simulink model "LKAS_with_MPC"  (R2021b)
settings: Solver=FixedStepAuto  StartTime=0.0  StopTime=20  FixedStep=0.1  MinStep=0.001  RelTol=1e-3
PostLoadFcn:
  | if exist('scenarioName','var')
  |   helperAEBSetUp(scenarioName)
  | else
  |   helperAEBSetUp()
  | end
undefined symbols (not defined in the file): A, B, C, D, Vx_const, X0, Y0, Yaw0
libraries: mpclib x1, drivingscenarioandsensors x1
CloseFcn:
  | helperAEBSetUp(true);
settings Model: Creator=user  LastModifiedBy=user
settings DataIOCC: SaveFormat=Array  SaveState=on

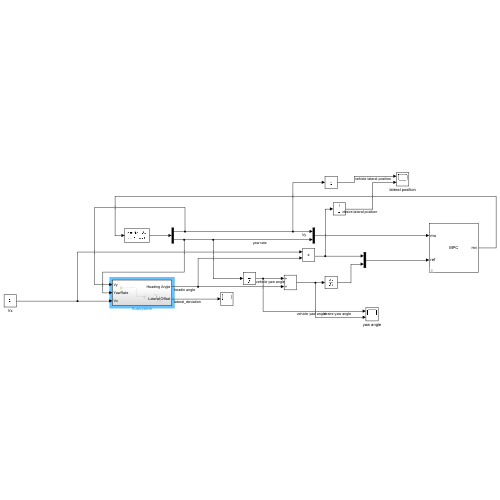
[thumbnail: Simulink's stored preview of the top-level diagram]
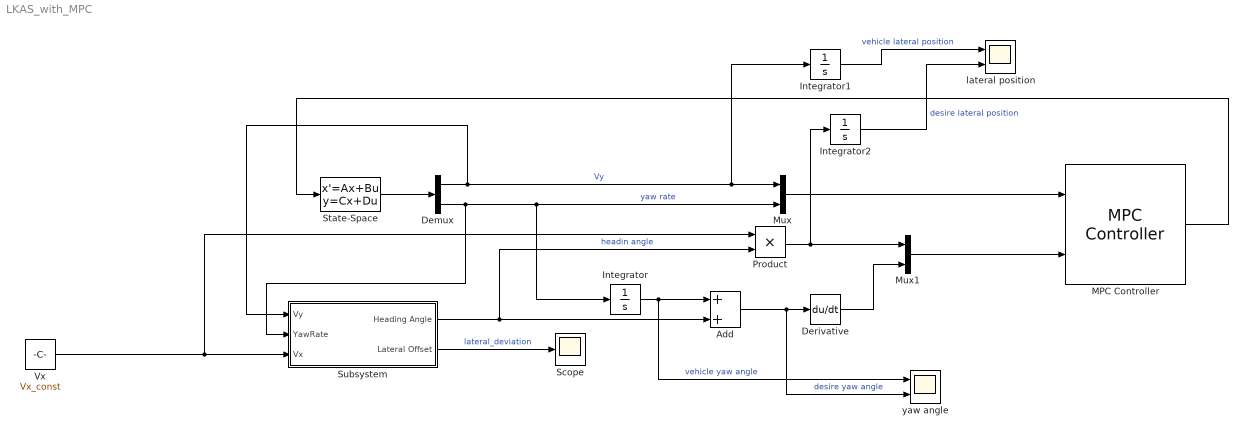
== system LKAS_with_MPC ==
  Add : Sum
  Demux : Demux  Outputs=2
  Derivative : Derivative
  Integrator : Integrator  InitialCondition=Yaw0
  Integrator1 : Integrator
  Integrator2 : Integrator
  MPC Controller : mpclib/MPC Controller  SCDEnableBlockLinearizationSpecification=on  mpcobj=mpc1  is_multiple=0  enable_value=0  return_u0=off  updateMPCinCallerWorkspace=on  md_inport=off  mv_inport=off  uref_inport=off  return_cost=off  return_mvseq=off  return_qpstatus=off  return_xseq=off  return_state=off  return_ovseq=off  state_inport=off  umin_inport=off  umax_inport=off  ymin_inport=off  ymax_inport=off  cc_inport=off  ywt_inport=off  uwt_inport=off  duwt_inport=off  rhoeps_inport=off  pm_inport=off  MaximumP=10  HorizonChoice=FixedHorizon  n_ts=0.1  n_p=20  n_mv=1  n_md=0  n_ud=0  n_mo=2  n_uo=0  BlockDataType=double  SampleTimeInherited=off  switch_inport=off
  Mux : Mux  Inputs=2
  Mux1 : Mux  Inputs=2
  Product : Product
  Scope : Scope
  State-Space : StateSpace  A=A  B=B  C=C  D=D  InitialCondition=0
  Subsystem : Subsystem
  Vx : Constant  Value=Vx_const
  lateral position : Scope  NumInputPorts=2
  yaw angle : Scope  NumInputPorts=2
  wires:
  Vx/1 -> Product/1, Subsystem/3(Vx)
  MPC Controller/1 -> State-Space/1
  Subsystem/1(Heading Angle) -> Product/2, Add/2  "headin angle"
  Integrator/1 -> yaw angle/1, Add/1  "vehicle yaw angle"
  Add/1 -> yaw angle/2, Derivative/1  "desire yaw angle"
  Mux1/1 -> MPC Controller/2
  Derivative/1 -> Mux1/2
  Subsystem/2(Lateral Offset) -> Scope/1  "lateral_deviation"
  Product/1 -> Integrator2/1, Mux1/1
  Mux/1 -> MPC Controller/1
  Demux/1 -> Integrator1/1, Mux/1, Subsystem/1(Vy)  "Vy"
  Demux/2 -> Subsystem/2(YawRate), Mux/2, Integrator/1  "yaw rate"
  State-Space/1 -> Demux/1
  Integrator1/1 -> lateral position/1  "vehicle lateral position"
  Integrator2/1 -> lateral position/2  "desire lateral position"

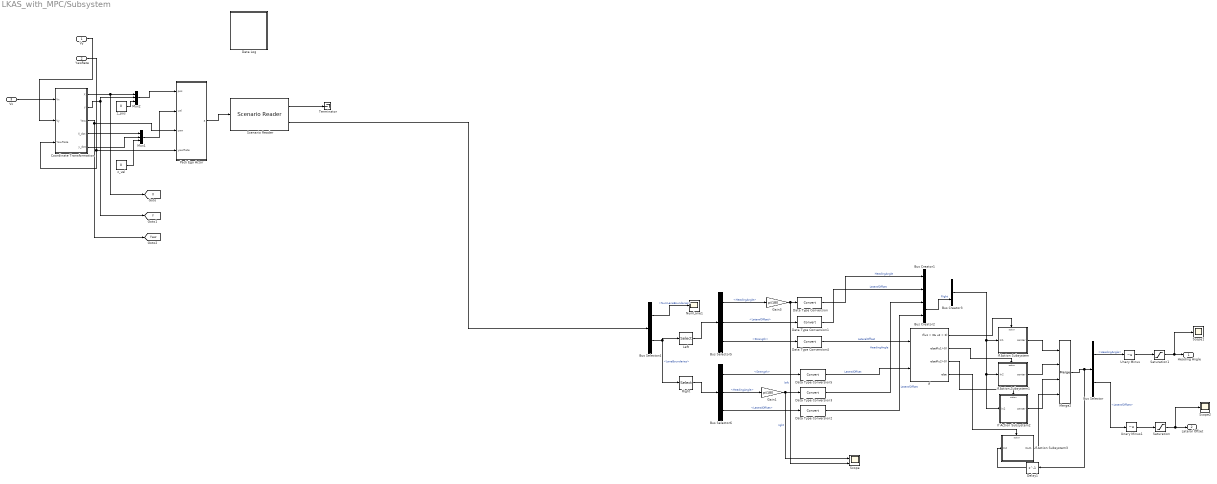
== system LKAS_with_MPC/Subsystem ==
  Vy : Inport
  YawRate : Inport  Port=2
  Vx : Inport  Port=3
  Bus Creator1 : BusCreator  Inputs=2
  Bus Creator2 : BusCreator  Inputs=2
  Bus Creator3 : BusCreator  Inputs=2
  Bus Selector : BusSelector  OutputSignals=HeadingAngle,LateralOffset
  Bus Selector4 : BusSelector  OutputSignals=NumLaneBoundaries,LaneBoundaries
  Bus Selector5 : BusSelector  OutputSignals=HeadingAngle,LateralOffset,Strength
  Bus Selector6 : BusSelector  OutputSignals=Strength,HeadingAngle,LateralOffset
  Coordinate Transformation : Subsystem
  Data Log : Subsystem
  Data Type Conversion{,1..5} (6 alike) : DataTypeConversion
  Delay1 : Delay  DelayLength=1
  Gain1 : Gain  Gain=pi/180
  Gain3 : Gain  Gain=pi/180
  If : If  NumInputs=2  IfExpression=u1 > 0& u2 > 0  ElseIfExpressions=u1>0, u2>0
  If Action Subsystem : Subsystem  TreatAsAtomicUnit=on
  If Action Subsystem1 : Subsystem  TreatAsAtomicUnit=on
  If Action Subsystem2 : Subsystem  TreatAsAtomicUnit=on
  If Action Subsystem3 : Subsystem  TreatAsAtomicUnit=on
  Left : Selector  InputPortWidth=2  IndexOptions=Index vector (dialog)  Indices=[1]  OutputSizes=1
  Merge2 : Merge  Inputs=4
  Mux1 : Mux  Inputs=3
  Mux2 : Mux  Inputs=3
  NumLane1 : Scope
  Pack Ego Actor : MATLAB Function  TreatAsAtomicUnit=on
  Right : Selector  InputPortWidth=2  IndexOptions=Index vector (dialog)  Indices=[2]  OutputSizes=1
  Saturation : Saturate
  Saturation1 : Saturate  UpperLimit=0.6  LowerLimit=-0.6
  Scenario Reader : drivingscenarioandsensors/Scenario Reader  ScenarioSource=From file  ScenarioFileName=C:\Users\user\Documents\MATLAB\Fproject\drivecurve.mat  ScenarioVariableName=scenario  OutputCoordinateSystem=Vehicle coordinates  EgoVehicleSource=Input port  EgoVehicleActorID=1  OrientVehiclesOnRoad=on  OutputEgoVehiclePose=off  OutputEgoVehicleState=off  SampleTime=0.1  LaneBoundaryOutput=Ego vehicle lane boundaries  LaneBoundaryDistance=0:0.5:9.5  LaneBoundaryLocation=Center of lane markings  BusNameSource=Auto  BusName=BusActors  BusNumActorsSource=Scenario  BusNumActors=100  BusName2Source=Auto  BusName2=BusLaneBoundaries  BusNumLaneBoundariesSource=Scenario  BusNumLaneBoundaries=10  BusName3Source=Auto  BusName3=BusEgoActor  BusName4Source=Auto  BusName4=BusEgoState  ShowCoordinateLabels=on  SimulateUsing=Interpreted execution
  Scope : Scope  NumInputPorts=2
  Scope1 : Scope
  Scope2 : Scope
  Terminator : Terminator
  Unary Minus : UnaryMinus
  Unary Minus1 : UnaryMinus
  z_pos : Constant  Value=0
  z_vel : Constant  Value=0
  Heading Angle : Outport  VectorParamsAs1DForOutWhenUnconnected=off
  Lateral Offset : Outport  Port=2  VectorParamsAs1DForOutWhenUnconnected=off
  tag scope: X=global, Y=global, Yaw=global
  wires:
  Coordinate Transformation/3(Yaw) -> Pack Ego Actor/3(yaw), [Yaw]
  YawRate/1 -> Pack Ego Actor/4(yawRate), Coordinate Transformation/3(YawRate)
  Coordinate Transformation/1(X) -> [X], Mux2/1
  Vy/1 -> Coordinate Transformation/2(Vy)
  z_pos/1 -> Mux2/3
  Coordinate Transformation/5(y_dot) -> Mux1/2
  Mux1/1 -> Pack Ego Actor/2(vel)
  Coordinate Transformation/4(X_dot) -> Mux1/1
  Scenario Reader/1 -> Terminator/1
  Mux2/1 -> Pack Ego Actor/1(pos)
  Coordinate Transformation/2(Y) -> [Y], Mux2/2
  z_vel/1 -> Mux1/3
  Vx/1 -> Coordinate Transformation/1(Vx)
  Data Type Conversion/1 -> Bus Creator1/1  "HeadingAngle"
  Bus Selector/2 -> Unary Minus1/1  "<LateralOffset>"
  If Action Subsystem/1(center) -> Merge2/1
  Bus Creator2/1 -> Bus Creator3/2  "Right"
  Bus Selector/1 -> Unary Minus/1  "<HeadingAngle>"
  Merge2/1 -> Delay1/1, Bus Selector/1
  Bus Selector6/2 -> Gain1/1  "<HeadingAngle>"
  Unary Minus1/1 -> Saturation/1
  Right/1 -> Bus Selector6/1
  Scenario Reader/2 -> Bus Selector4/1
  If/4 -> If Action Subsystem3/Action
  Bus Creator3/1 -> If Action Subsystem2/1(In2), If Action Subsystem1/1(In2), If Action Subsystem/1(In1)
  If Action Subsystem1/1(center) -> Merge2/2
  Delay1/1 -> If Action Subsystem3/1(In2)
  If Action Subsystem3/1(Out1) -> Merge2/4
  Saturation1/1 -> Scope1/1, Heading Angle/1
  Bus Selector5/1 -> Gain3/1  "<HeadingAngle>"
  If/2 -> If Action Subsystem1/Action
  Data Type Conversion4/1 -> If/1  "LateralOffset"
  Bus Selector6/1 -> Data Type Conversion5/1  "<Strength>"
  If/1 -> If Action Subsystem/Action
  Data Type Conversion3/1 -> Bus Creator2/1  "HeadingAngle"
  Data Type Conversion5/1 -> If/2  "LateralOffset"
  Saturation/1 -> Scope2/1, Lateral Offset/1
  If/3 -> If Action Subsystem2/Action
  Unary Minus/1 -> Saturation1/1
  If Action Subsystem2/1(center) -> Merge2/3
  Bus Selector4/2 -> Left/1, Right/1  "<LaneBoundaries>"
  Gain1/1 -> Scope/1, Data Type Conversion3/1  "right"
  Left/1 -> Bus Selector5/1
  Data Type Conversion2/1 -> Bus Creator2/2  "LateralOffset"
  Bus Selector4/1 -> NumLane1/1  "<NumLaneBoundaries>"
  Gain3/1 -> Scope/2, Data Type Conversion/1  "left"
  Bus Selector5/3 -> Data Type Conversion4/1  "<Strength>"
  Data Type Conversion1/1 -> Bus Creator1/2  "LateralOffset"
  Bus Selector6/3 -> Data Type Conversion2/1  "<LateralOffset>"
  Bus Selector5/2 -> Data Type Conversion1/1  "<LateralOffset>"
  Pack Ego Actor/1(a) -> Scenario Reader/1

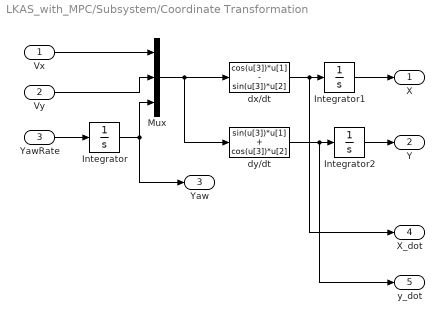
== system LKAS_with_MPC/Subsystem/Coordinate Transformation ==
  Vx : Inport
  Vy : Inport  Port=2
  YawRate : Inport  Port=3
  Integrator : Integrator  InitialCondition=Yaw0
  Integrator1 : Integrator  InitialCondition=X0
  Integrator2 : Integrator  InitialCondition=Y0
  Mux : Mux  Inputs=3
  dx/dt : Fcn  Expr=cos(u[3])*u[1] - sin(u[3])*u[2]
  dy/dt : Fcn  Expr=sin(u[3])*u[1] + cos(u[3])*u[2]
  X : Outport
  Y : Outport  Port=2
  Yaw : Outport  Port=3
  X_dot : Outport  Port=4
  y_dot : Outport  Port=5
  wires:
  YawRate/1 -> Integrator/1
  Vx/1 -> Mux/1
  Vy/1 -> Mux/2
  Integrator/1 -> Mux/3, Yaw/1
  Mux/1 -> dx/dt/1, dy/dt/1
  dx/dt/1 -> X_dot/1, Integrator1/1
  Integrator1/1 -> X/1
  dy/dt/1 -> y_dot/1, Integrator2/1
  Integrator2/1 -> Y/1

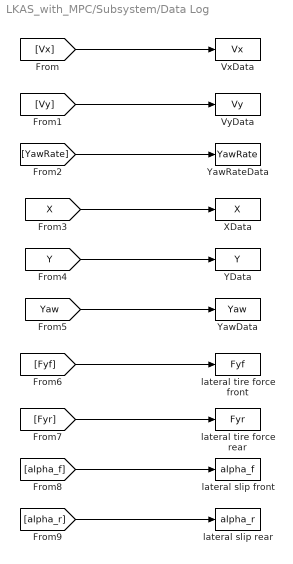
== system LKAS_with_MPC/Subsystem/Data Log ==
  VxData : ToWorkspace  VariableName=Vx  SampleTime=-1
  VyData : ToWorkspace  VariableName=Vy  SampleTime=-1
  XData : ToWorkspace  VariableName=X  SampleTime=-1
  YData : ToWorkspace  VariableName=Y  SampleTime=-1
  YawData : ToWorkspace  VariableName=Yaw  SampleTime=-1
  YawRateData : ToWorkspace  VariableName=YawRate  SampleTime=-1
  lateral slip front : ToWorkspace  VariableName=alpha_f  SampleTime=-1
  lateral slip rear : ToWorkspace  VariableName=alpha_r  SampleTime=-1
  lateral tire force front : ToWorkspace  VariableName=Fyf  SampleTime=-1
  lateral tire force rear : ToWorkspace  VariableName=Fyr  SampleTime=-1
  wires:
  [Vx] -> VxData/1
  [Vy] -> VyData/1
  [YawRate] -> YawRateData/1
  [X] -> XData/1
  [Y] -> YData/1
  [Yaw] -> YawData/1
  [Fyf] -> lateral tire force front/1
  [Fyr] -> lateral tire force rear/1
  [alpha_f] -> lateral slip front/1
  [alpha_r] -> lateral slip rear/1

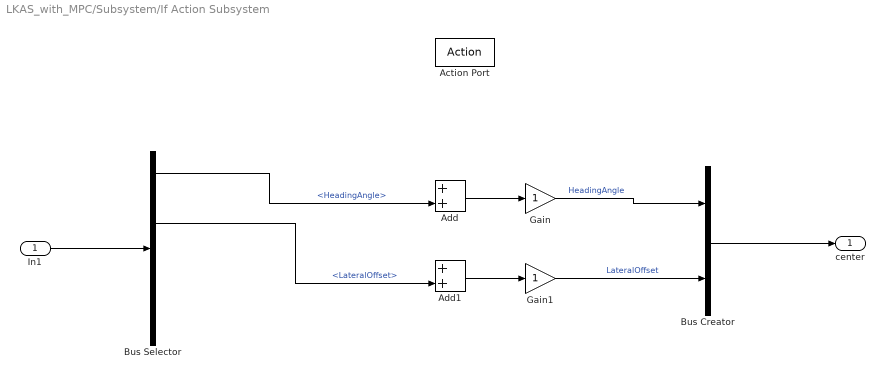
== system LKAS_with_MPC/Subsystem/If Action Subsystem ==
  In1 : Inport
  Action Port : ActionPort  ActionPortLabel=if(u1 > 0& u2 > 0)
  Add : Sum
  Add1 : Sum
  Bus Creator : BusCreator  Inputs=2
  Bus Selector : BusSelector  OutputSignals=Right.HeadingAngle,Right.LateralOffset,Right.HeadingAngle,Right.LateralOffset
  Gain : Gain
  Gain1 : Gain
  center : Outport
  wires:
  In1/1 -> Bus Selector/1
  ? -> Add/1  "<HeadingAngle>"
  Add/1 -> Gain/1
  Add1/1 -> Gain1/1
  Gain/1 -> Bus Creator/1  "HeadingAngle"
  Gain1/1 -> Bus Creator/2  "LateralOffset"
  ? -> Add1/1  "<LateralOffset>"
  Bus Selector/1 -> Add/2  "<HeadingAngle>"
  Bus Selector/2 -> Add1/2  "<LateralOffset>"
  Bus Creator/1 -> center/1

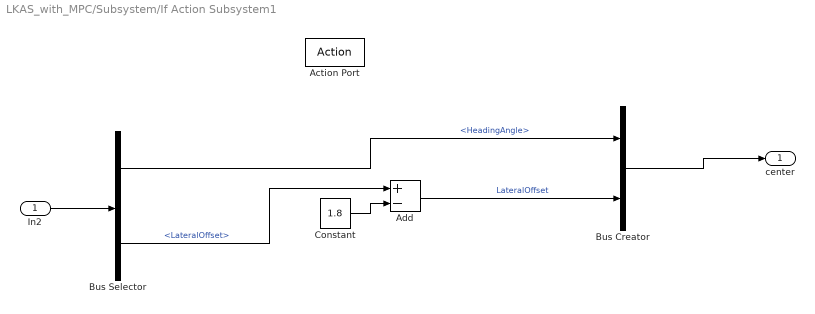
== system LKAS_with_MPC/Subsystem/If Action Subsystem1 ==
  In2 : Inport
  Action Port : ActionPort  ActionPortLabel=elseif(u1>0)
  Add : Sum  Inputs=+-
  Bus Creator : BusCreator  Inputs=2
  Bus Selector : BusSelector  OutputSignals=Right.HeadingAngle,Right.LateralOffset
  Constant : Constant  Value=1.8
  center : Outport
  wires:
  In2/1 -> Bus Selector/1
  Bus Selector/1 -> Bus Creator/1  "<HeadingAngle>"
  Constant/1 -> Add/2
  Add/1 -> Bus Creator/2  "LateralOffset"
  Bus Selector/2 -> Add/1  "<LateralOffset>"
  Bus Creator/1 -> center/1

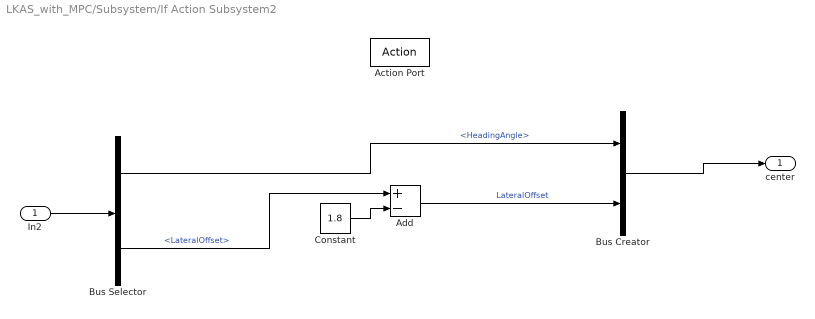
== system LKAS_with_MPC/Subsystem/If Action Subsystem2 ==
  In2 : Inport
  Action Port : ActionPort  ActionPortLabel=elseif( u2>0)
  Add : Sum  Inputs=+-
  Bus Creator : BusCreator  Inputs=2
  Bus Selector : BusSelector  OutputSignals=Right.HeadingAngle,Right.LateralOffset
  Constant : Constant  Value=1.8
  center : Outport
  wires:
  In2/1 -> Bus Selector/1
  Bus Selector/2 -> Add/1  "<LateralOffset>"
  Constant/1 -> Add/2
  Bus Selector/1 -> Bus Creator/1  "<HeadingAngle>"
  Bus Creator/1 -> center/1
  Add/1 -> Bus Creator/2  "LateralOffset"

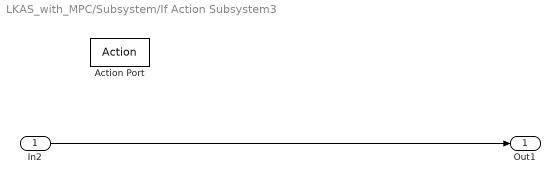
== system LKAS_with_MPC/Subsystem/If Action Subsystem3 ==
  In2 : Inport
  Action Port : ActionPort  ActionPortLabel=else
  Out1 : Outport
  wires:
  In2/1 -> Out1/1

== matlab function LKAS_with_MPC/Subsystem/Pack Ego Actor ==
  data: pos input; a output Bus: BusActors1Actors size=1; vel input; yaw input; yawRate input
function a = packEgo(pos,vel,yaw,yawRate)
% Pack ego information into a single ego actor bus
%
% Imoprtant note:
% Output is a bus of type BusActorsActors. This is the same bus used by the
% Scenario Reader to output an individual actor. If you change the
% output bus name of Scenario Reader change the output bus name here
% as well by clicking on 'Edit Data' in the menu above.

a = struct(...
    'ActorID',2,...
    'Position', [pos(1) pos(2) 0], ...
    'Velocity', [vel(1) vel(2) 0], ...
    'Roll', 0, ...
    'Pitch', 0, ...
    'Yaw', yaw, ...
    'AngularVelocity', [0 0 yawRate]);
